simulink model "main_WU_motion"  (R2023a)
settings: Solver=VariableStepAuto  StartTime=0.0  StopTime=3.88  RelTol=1e-9  AbsTol=1e-9  EnableMultiTasking=on
values from neighbouring files (symbols this model uses):
  a_el = [r_ej,h_ej,r_ej]    [data.m]    (also in fo_python_to_matlab.m = [ax,ay,az])
  akt_GH = rand(1,13)*1    [inverse_dynamics.m]    (also in odvozeni_svaly.m = sym('akt_GH',[1 N_GH]))
  akt_ST = rand(1,13)*1    [inverse_dynamics.m]    (also in odvozeni_svaly.m = sym('akt_ST',[1 N_ST]))
  ccom = [-0.0110972, 0.00637508, 0.0541825]    [data.m]    (also in fo_python_to_matlab.m = [ccomx, ccomy, ccomz]; mm_python_to_matlab.m = [ccomx, ccomy, ccomz])
  cI = [5.75482e-05, 6.05521e-05, 1.05345e-05,-1.27405e-05, 1.65861e-05, 4.50136e-06]    [data.m]    (also in mm_python_to_matlab.m = [cixx, ciyy, cizz, cixy, ciyz, cizx])
  cont1 = [-0.083529 -0.01368 -0.098954]-scom    [data.m]    (also in fo_python_to_matlab.m = [x_cont1,y_cont1,z_cont1])
  cont2 = [-0.105456 -0.125076 -0.075251]-scom    [data.m]    (also in fo_python_to_matlab.m = [x_cont2,y_cont2,z_cont2])
  cont_params = [k_contact, eps]    [data.m]    (also in fo_python_to_matlab.m)
  Glenohumeral_F0M = str2double(table2array(GH(:,2)))'    [data.m]
  Glenohumeral_l0 = str2double(table2array(GH(:,3)))'    [data.m]
  h_ej = 0.15    [data.m]
  hcom = [0.000389382, -0.116338, -0.00231072]    [data.m]    (also in fo_python_to_matlab.m = [hcomx, hcomy, hcomz]; mm_python_to_matlab.m = [hcomx, hcomy, hcomz])
  hI = [0.00326632, 4.34807e-05, 0.00325004,-0.000136456, -1.30958e-06, -1.14964e-05]    [data.m]    (also in mm_python_to_matlab.m = [hixx, hiyy, hizz, hixy, hiyz, hizx])
  initialConditions = zeros(1,18)    [inverse_dynamics.m]
  k_contact = 0    [data.m]
  m = [0.0370005,0.12759,0.26363]    [data.m]    (also in fo_python_to_matlab.m = [c_m,s_m,h_m]; mm_python_to_matlab.m = [c_m,s_m,h_m])
  m_el = [x_ej,y_ej,z_ej]    [data.m]    (also in fo_python_to_matlab.m = [mx, my, mz])
  p = [c,k,g]    [data.m]    (also in fo_python_to_matlab.m)
  r_ej = 0.088    [data.m]
  Scapulothoracic_F0M = str2double(table2array(ST(:,2)))'    [data.m]
  Scapulothoracic_l0 = str2double(table2array(ST(:,3)))'    [data.m]
  scom = [-0.0512948, -0.0367122, -0.0430756]    [data.m]    (also in fo_python_to_matlab.m = [scomx, scomy, scomz]; mm_python_to_matlab.m = [scomx, scomy, scomz])
  sI = [0.00020065, 0.000202939, 0.000227237,-4.55661e-05, -7.53511e-05, -7.42694e-05]    [data.m]    (also in mm_python_to_matlab.m = [sixx, siyy, sizz, sixy, siyz, sizx])
  T_c = [-0.01433 0.02007 0.135535]    [data.m]    (also in fo_python_to_matlab.m = [T_cx,T_cy,T_cz]; mm_python_to_matlab.m = [T_cx,T_cy,T_cz]; odvozeni_svaly.m)
  T_d = 1e-20    [data.m]
  T_s = [-0.00955 -0.034 0.009]    [data.m]    (also in fo_python_to_matlab.m = [T_sx,T_sy,T_sz]; mm_python_to_matlab.m = [T_sx,T_sy,T_sz]; odvozeni_svaly.m)
  T_t = [0.006325 0.00693 0.025465]    [data.m]    (also in fo_python_to_matlab.m = [T_tx, T_ty, T_tz]; odvozeni_svaly.m)
  x_ej = -0.03    [data.m]
  y_ej = -0.1    [data.m]
  z_ej = 0.05    [data.m]
undefined symbols (not defined in the file or in its folder): phi_0, r_0, r_10, r_20, X, Y, Z
libraries: sm_lib x165, nesl_utility x96
(part 5 of 5)

== system main_WU_motion/scapulohumeral_rhythm/2_points_contact/ellipsoidal_joint_2 ==
  PS-Simulink Converter : nesl_utility/PS-Simulink Converter  PhysicalDomain=network_engine_domain  SubClassName=ps_output  LeftPortType=input  RightPortType=output  PseudoPeriodic=off  Frequencies=[]  VectorFormat=inherit  Unit=inherit  AffineConversion=off
  Simulink-PS Converter : nesl_utility/Simulink-PS Converter  PhysicalDomain=network_engine_domain  SubClassName=ps_input  LeftPortType=input  RightPortType=output  PseudoPeriodic=off  Frequencies=[]  NoiseDistribution=none  NoiseParameters=[]  Unit=1  AffineConversion=off  FilteringAndDerivatives=filter  SimscapeFilterOrder=2  InputFilterTimeConstant=0.001  UdotUserProvided=0
  axis : sm_lib/Joints/Revolute Joint  JointMode=Normal  SenseConstraintForce=off  SenseConstraintForceX=off  SenseConstraintForceY=off  SenseConstraintForceZ=off  SenseConstraintTorque=off  SenseConstraintTorqueX=off  SenseConstraintTorqueY=off  SenseConstraintTorqueZ=off  SenseTotalForce=off  SenseTotalForceX=off  SenseTotalForceY=off  SenseTotalForceZ=off  SenseTotalTorque=off  SenseTotalTorqueX=off  SenseTotalTorqueY=off  SenseTotalTorqueZ=off  CompositeWrenchDir=FollowerOnBase  CompositeWrenchFrame=BaseFrame  EquilibriumPosition=0  EquilibriumPositionUnits=deg  SpringStiffness=0  SpringStiffnessUnits=N*m/deg  DampingCoefficient=0  DampingCoefficientUnits=N*m/(deg/s)  TorqueActuationMode=NoTorque  MotionActuationMode=ComputedMotion  SensePosition=off  SenseVelocity=off  SenseAcceleration=off  SenseTorqueForce=off  SenseLowerLimitTorqueForce=off  SenseUpperLimitTorqueForce=off  LowerLimitSpecify=off  LowerLimitBound=-90  LowerLimitBoundUnits=deg  LowerLimitStiffness=1e4  LowerLimitStiffnessUnits=N*m/deg  LowerLimitDamping=10  LowerLimitDampingUnits=N*m/(deg/s)  LowerLimitTransitionRegionWidth=0.1  LowerLimitTransitionRegionWidthUnits=deg  UpperLimitSpecify=off  UpperLimitBound=90  UpperLimitBoundUnits=deg  UpperLimitStiffness=1e4  UpperLimitStiffnessUnits=N*m/deg  UpperLimitDamping=10  UpperLimitDampingUnits=N*m/(deg/s)  UpperLimitTransitionRegionWidth=0.1  UpperLimitTransitionRegionWidthUnits=deg  PositionTargetSpecify=on  PositionTargetPriority=High  PositionTargetValue=phi_20  PositionTargetValueUnits=rad  VelocityTargetSpecify=on  VelocityTargetPriority=High  VelocityTargetValue=0  VelocityTargetValueUnits=rad/s
  delay_r : TransportDelay  DelayTime=T_d  InitialOutput=r_20
  h : sm_lib/Joints/Prismatic Joint  JointMode=Normal  SenseConstraintForce=off  SenseConstraintForceX=off  SenseConstraintForceY=off  SenseConstraintForceZ=off  SenseConstraintTorque=off  SenseConstraintTorqueX=off  SenseConstraintTorqueY=off  SenseConstraintTorqueZ=off  SenseTotalForce=off  SenseTotalForceX=off  SenseTotalForceY=off  SenseTotalForceZ=off  SenseTotalTorque=off  SenseTotalTorqueX=off  SenseTotalTorqueY=off  SenseTotalTorqueZ=off  CompositeWrenchDir=FollowerOnBase  CompositeWrenchFrame=BaseFrame  EquilibriumPosition=0  EquilibriumPositionUnits=m  SpringStiffness=0  SpringStiffnessUnits=N/m  DampingCoefficient=0  DampingCoefficientUnits=N/(m/s)  TorqueActuationMode=NoTorque  MotionActuationMode=ComputedMotion  SensePosition=on  SenseVelocity=off  SenseAcceleration=off  SenseTorqueForce=off  SenseLowerLimitTorqueForce=off  SenseUpperLimitTorqueForce=off  LowerLimitSpecify=on  LowerLimitBound=h_min  LowerLimitBoundUnits=m  LowerLimitStiffness=1e6  LowerLimitStiffnessUnits=N/m  LowerLimitDamping=1e3  LowerLimitDampingUnits=N/(m/s)  LowerLimitTransitionRegionWidth=1e-4  LowerLimitTransitionRegionWidthUnits=m  UpperLimitSpecify=on  UpperLimitBound=h_max  UpperLimitBoundUnits=m  UpperLimitStiffness=1e6  UpperLimitStiffnessUnits=N/m  UpperLimitDamping=1e3  UpperLimitDampingUnits=N/(m/s)  UpperLimitTransitionRegionWidth=1e-4  UpperLimitTransitionRegionWidthUnits=m  PositionTargetSpecify=on  PositionTargetPriority=High  PositionTargetValue=h_20  PositionTargetValueUnits=m  VelocityTargetSpecify=on  VelocityTargetPriority=High  VelocityTargetValue=0  VelocityTargetValueUnits=m/s
  r : sm_lib/Joints/Prismatic Joint  JointMode=Normal  SenseConstraintForce=off  SenseConstraintForceX=off  SenseConstraintForceY=off  SenseConstraintForceZ=off  SenseConstraintTorque=off  SenseConstraintTorqueX=off  SenseConstraintTorqueY=off  SenseConstraintTorqueZ=off  SenseTotalForce=off  SenseTotalForceX=off  SenseTotalForceY=off  SenseTotalForceZ=off  SenseTotalTorque=off  SenseTotalTorqueX=off  SenseTotalTorqueY=off  SenseTotalTorqueZ=off  CompositeWrenchDir=FollowerOnBase  CompositeWrenchFrame=BaseFrame  EquilibriumPosition=0  EquilibriumPositionUnits=m  SpringStiffness=0  SpringStiffnessUnits=N/m  DampingCoefficient=0  DampingCoefficientUnits=N/(m/s)  TorqueActuationMode=ComputedTorque  MotionActuationMode=InputMotion  SensePosition=off  SenseVelocity=off  SenseAcceleration=off  SenseTorqueForce=off  SenseLowerLimitTorqueForce=off  SenseUpperLimitTorqueForce=off  LowerLimitSpecify=off  LowerLimitBound=-1  LowerLimitBoundUnits=m  LowerLimitStiffness=1e6  LowerLimitStiffnessUnits=N/m  LowerLimitDamping=1e3  LowerLimitDampingUnits=N/(m/s)  LowerLimitTransitionRegionWidth=1e-4  LowerLimitTransitionRegionWidthUnits=m  UpperLimitSpecify=off  UpperLimitBound=1  UpperLimitBoundUnits=m  UpperLimitStiffness=1e6  UpperLimitStiffnessUnits=N/m  UpperLimitDamping=1e3  UpperLimitDampingUnits=N/(m/s)  UpperLimitTransitionRegionWidth=1e-4  UpperLimitTransitionRegionWidthUnits=m  PositionTargetSpecify=on  PositionTargetPriority=Low  PositionTargetValue=r_20  PositionTargetValueUnits=m  VelocityTargetSpecify=on  VelocityTargetPriority=Low  VelocityTargetValue=0  VelocityTargetValueUnits=m/s
  r = fcn(h) : MATLAB Function  TreatAsAtomicUnit=on
  rot_-x_90 : sm_lib/Frames and Transforms/Rigid Transform  TranslationMethod=None  TranslationStandardOffset=0  TranslationStandardOffsetUnits=m  TranslationStandardAxis=+Z  TranslationCartesianOffset=[0 0 0]  TranslationCartesianOffsetUnits=m  TranslationROffset=0  TranslationROffsetUnits=m  TranslationZOffset=0  TranslationZOffsetUnits=m  TranslationThetaOffset=0  TranslationThetaOffsetUnits=deg  RotationMethod=StandardAxis  RotationAngleUnits=deg  RotationStandardAxis=-X  RotationAngle=90  RotationArbitraryAxis=[0 0 1]  FollAlignAxisA=+X  BaseAlignAxisA=+Y  FollAlignAxisB=+Y  BaseAlignAxisB=+Z  RotationSequenceAxes=FollowerAxes  RotationSequence=XYX  RotationSequenceAngles=[0 0 0]  RotationSequenceAnglesUnits=deg  RotationMatrix=[1 0 0; 0 1 0; 0 0 1]  Quaternion=[1 0 0 0]
  rot_-y_90 : sm_lib/Frames and Transforms/Rigid Transform  TranslationMethod=None  TranslationStandardOffset=0  TranslationStandardOffsetUnits=m  TranslationStandardAxis=+Z  TranslationCartesianOffset=[0 0 0]  TranslationCartesianOffsetUnits=m  TranslationROffset=0  TranslationROffsetUnits=m  TranslationZOffset=0  TranslationZOffsetUnits=m  TranslationThetaOffset=0  TranslationThetaOffsetUnits=deg  RotationMethod=StandardAxis  RotationAngleUnits=deg  RotationStandardAxis=-Y  RotationAngle=90  RotationArbitraryAxis=[0 0 1]  FollAlignAxisA=+X  BaseAlignAxisA=+Y  FollAlignAxisB=+Y  BaseAlignAxisB=+Z  RotationSequenceAxes=FollowerAxes  RotationSequence=XYX  RotationSequenceAngles=[0 0 0]  RotationSequenceAnglesUnits=deg  RotationMatrix=[1 0 0; 0 1 0; 0 0 1]  Quaternion=[1 0 0 0]
  scp_h : Scope
  scp_r : Scope
  B : PMIOPort  Side=Left
  F : PMIOPort  Port=2  Side=Right
  wires:
  PS-Simulink Converter/1 -> r = fcn(h)/1(h), scp_h/1
  delay_r/1 -> scp_r/1, Simulink-PS Converter/1
  r = fcn(h)/1(r) -> delay_r/1
  connections:
  rot_-x_90/LConn1 -- B/RConn1
  axis/LConn1 -- rot_-x_90/RConn1
  h/RConn2 -- PS-Simulink Converter/LConn1
  Simulink-PS Converter/RConn1 -- r/LConn2
  r/LConn1 -- rot_-y_90/RConn1
  F/RConn1 -- r/RConn1
  h/RConn1 -- rot_-y_90/LConn1
  h/LConn1 -- axis/RConn1

== system main_WU_motion/scapulohumeral_rhythm/2_points_contact/tools ==
  In1 : Inport
  cartensian_X : Subsystem

== system main_WU_motion/scapulohumeral_rhythm/Subsystem/point 1 ==
  External Force and Torque : sm_lib/Forces and Torques/External Force and Torque  ForceResolutionFrame=World  EnableForceX=on  EnableForceY=on  EnableForceZ=on  EnableForce=off  TorqueResolutionFrame=AttachedFrame  EnableTorqueX=off  EnableTorqueY=off  EnableTorqueZ=off  EnableTorque=off
  F : MATLAB Function  TreatAsAtomicUnit=on
  Mux : Mux  Inputs=3
  Mux1 : Mux  Inputs=3
  PS-Simulink Converter : nesl_utility/PS-Simulink Converter  PhysicalDomain=network_engine_domain  SubClassName=ps_output  LeftPortType=input  RightPortType=output  PseudoPeriodic=off  Frequencies=[]  VectorFormat=inherit  Unit=inherit  AffineConversion=off
  PS-Simulink Converter1 : nesl_utility/PS-Simulink Converter  PhysicalDomain=network_engine_domain  SubClassName=ps_output  LeftPortType=input  RightPortType=output  PseudoPeriodic=off  Frequencies=[]  VectorFormat=inherit  Unit=inherit  AffineConversion=off
  PS-Simulink Converter2 : nesl_utility/PS-Simulink Converter  PhysicalDomain=network_engine_domain  SubClassName=ps_output  LeftPortType=input  RightPortType=output  PseudoPeriodic=off  Frequencies=[]  VectorFormat=inherit  Unit=inherit  AffineConversion=off
  "S_1 -> S" : sm_lib/Frames and Transforms/Rigid Transform  TranslationMethod=Cartesian  TranslationStandardOffset=0  TranslationStandardOffsetUnits=m  TranslationStandardAxis=+Z  TranslationCartesianOffset=cont1  TranslationCartesianOffsetUnits=m  TranslationROffset=0  TranslationROffsetUnits=m  TranslationZOffset=0  TranslationZOffsetUnits=m  TranslationThetaOffset=0  TranslationThetaOffsetUnits=deg  RotationMethod=None  RotationAngleUnits=deg  RotationStandardAxis=+Z  RotationAngle=0.0  RotationArbitraryAxis=[0 0 1]  FollAlignAxisA=+X  BaseAlignAxisA=+Y  FollAlignAxisB=+Y  BaseAlignAxisB=+Z  RotationSequenceAxes=FollowerAxes  RotationSequence=XYX  RotationSequenceAngles=[0 0 0]  RotationSequenceAnglesUnits=deg  RotationMatrix=[1 0 0; 0 1 0; 0 0 1]  Quaternion=[1 0 0 0]
  Scope : Scope
  Simulink-PS Converter : nesl_utility/Simulink-PS Converter  PhysicalDomain=network_engine_domain  SubClassName=ps_input  LeftPortType=input  RightPortType=output  PseudoPeriodic=off  Frequencies=[]  NoiseDistribution=none  NoiseParameters=[]  Unit=1  AffineConversion=off  FilteringAndDerivatives=provide  SimscapeFilterOrder=1  InputFilterTimeConstant=0.001  UdotUserProvided=0
  Simulink-PS Converter1 : nesl_utility/Simulink-PS Converter  PhysicalDomain=network_engine_domain  SubClassName=ps_input  LeftPortType=input  RightPortType=output  PseudoPeriodic=off  Frequencies=[]  NoiseDistribution=none  NoiseParameters=[]  Unit=1  AffineConversion=off  FilteringAndDerivatives=provide  SimscapeFilterOrder=1  InputFilterTimeConstant=0.001  UdotUserProvided=0
  Simulink-PS Converter2 : nesl_utility/Simulink-PS Converter  PhysicalDomain=network_engine_domain  SubClassName=ps_input  LeftPortType=input  RightPortType=output  PseudoPeriodic=off  Frequencies=[]  NoiseDistribution=none  NoiseParameters=[]  Unit=1  AffineConversion=off  FilteringAndDerivatives=provide  SimscapeFilterOrder=1  InputFilterTimeConstant=0.001  UdotUserProvided=0
  Terminator : Terminator
  Transform Sensor : sm_lib/Frames and Transforms/Transform Sensor  MeasurementFrame=World  RotationSequence=XYX  SenseAngle=off  SenseAxis=off  SenseQ=off  SenseR=off  SenseRotationSequence=off  SenseOmegaX=off  SenseOmegaY=off  SenseOmegaZ=off  SenseQDot=off  SenseRDot=off  SenseRotationSequenceDot=off  SenseAlphaX=off  SenseAlphaY=off  SenseAlphaZ=off  SenseQDDot=off  SenseRDDot=off  SenseX=on  SenseY=on  SenseZ=on  SenseRad=off  SenseAzim=off  SenseDist=off  SenseInc=off  SenseXDot=off  SenseYDot=off  SenseZDot=off  SenseRadDot=off  SenseAzimDot=off  SenseDistDot=off  SenseIncDot=off  SenseXDDot=off  SenseYDDot=off  SenseZDDot=off  SenseRadDDot=off  SenseAzimDDot=off  SenseDistDDot=off  SenseIncDDot=off
  Frame : PMIOPort  Side=Left
  Contact point1 : PMIOPort  Port=2  Side=Right
  contact point 1 force : Outport
  wires:
  PS-Simulink Converter2/1 -> Mux1/3, F/3(z)
  F/3(Fz) -> contact point 1 force/1, Simulink-PS Converter2/1, Mux/3  "z"
  PS-Simulink Converter1/1 -> Mux1/2, F/2(y)
  F/1(Fx) -> Simulink-PS Converter/1, Mux/1  "x"
  F/2(Fy) -> Simulink-PS Converter1/1, Mux/2  "y"
  PS-Simulink Converter/1 -> Mux1/1, F/1(x)
  Mux1/1 -> Scope/1
  Mux/1 -> Terminator/1
  connections:
  External Force and Torque/LConn2 -- Simulink-PS Converter1/RConn1
  Transform Sensor/RConn4 -- PS-Simulink Converter2/LConn1
  Transform Sensor/RConn2 -- PS-Simulink Converter/LConn1
  Transform Sensor/LConn1 -- Frame/RConn1
  Simulink-PS Converter/RConn1 -- External Force and Torque/LConn1
  Transform Sensor/RConn3 -- PS-Simulink Converter1/LConn1
  Simulink-PS Converter2/RConn1 -- External Force and Torque/LConn3
  External Force and Torque/RConn1 -- "S_1 -> S"/RConn1 -- Transform Sensor/RConn1
  "S_1 -> S"/LConn1 -- Contact point1/RConn1

== system main_WU_motion/scapulohumeral_rhythm/Subsystem/point 2 ==
  External Force and Torque : sm_lib/Forces and Torques/External Force and Torque  ForceResolutionFrame=World  EnableForceX=on  EnableForceY=on  EnableForceZ=on  EnableForce=off  TorqueResolutionFrame=AttachedFrame  EnableTorqueX=off  EnableTorqueY=off  EnableTorqueZ=off  EnableTorque=off
  F : MATLAB Function  TreatAsAtomicUnit=on
  Mux : Mux  Inputs=3
  Mux1 : Mux  Inputs=3
  PS-Simulink Converter : nesl_utility/PS-Simulink Converter  PhysicalDomain=network_engine_domain  SubClassName=ps_output  LeftPortType=input  RightPortType=output  PseudoPeriodic=off  Frequencies=[]  VectorFormat=inherit  Unit=inherit  AffineConversion=off
  PS-Simulink Converter1 : nesl_utility/PS-Simulink Converter  PhysicalDomain=network_engine_domain  SubClassName=ps_output  LeftPortType=input  RightPortType=output  PseudoPeriodic=off  Frequencies=[]  VectorFormat=inherit  Unit=inherit  AffineConversion=off
  PS-Simulink Converter2 : nesl_utility/PS-Simulink Converter  PhysicalDomain=network_engine_domain  SubClassName=ps_output  LeftPortType=input  RightPortType=output  PseudoPeriodic=off  Frequencies=[]  VectorFormat=inherit  Unit=inherit  AffineConversion=off
  "S_2 -> S" : sm_lib/Frames and Transforms/Rigid Transform  TranslationMethod=Cartesian  TranslationStandardOffset=0  TranslationStandardOffsetUnits=m  TranslationStandardAxis=+Z  TranslationCartesianOffset=cont2  TranslationCartesianOffsetUnits=m  TranslationROffset=0  TranslationROffsetUnits=m  TranslationZOffset=0  TranslationZOffsetUnits=m  TranslationThetaOffset=0  TranslationThetaOffsetUnits=deg  RotationMethod=None  RotationAngleUnits=deg  RotationStandardAxis=+Z  RotationAngle=0.0  RotationArbitraryAxis=[0 0 1]  FollAlignAxisA=+X  BaseAlignAxisA=+Y  FollAlignAxisB=+Y  BaseAlignAxisB=+Z  RotationSequenceAxes=FollowerAxes  RotationSequence=XYX  RotationSequenceAngles=[0 0 0]  RotationSequenceAnglesUnits=deg  RotationMatrix=[1 0 0; 0 1 0; 0 0 1]  Quaternion=[1 0 0 0]
  Scope : Scope
  Simulink-PS Converter : nesl_utility/Simulink-PS Converter  PhysicalDomain=network_engine_domain  SubClassName=ps_input  LeftPortType=input  RightPortType=output  PseudoPeriodic=off  Frequencies=[]  NoiseDistribution=none  NoiseParameters=[]  Unit=1  AffineConversion=off  FilteringAndDerivatives=provide  SimscapeFilterOrder=1  InputFilterTimeConstant=0.001  UdotUserProvided=0
  Simulink-PS Converter1 : nesl_utility/Simulink-PS Converter  PhysicalDomain=network_engine_domain  SubClassName=ps_input  LeftPortType=input  RightPortType=output  PseudoPeriodic=off  Frequencies=[]  NoiseDistribution=none  NoiseParameters=[]  Unit=1  AffineConversion=off  FilteringAndDerivatives=provide  SimscapeFilterOrder=1  InputFilterTimeConstant=0.001  UdotUserProvided=0
  Simulink-PS Converter2 : nesl_utility/Simulink-PS Converter  PhysicalDomain=network_engine_domain  SubClassName=ps_input  LeftPortType=input  RightPortType=output  PseudoPeriodic=off  Frequencies=[]  NoiseDistribution=none  NoiseParameters=[]  Unit=1  AffineConversion=off  FilteringAndDerivatives=provide  SimscapeFilterOrder=1  InputFilterTimeConstant=0.001  UdotUserProvided=0
  Transform Sensor : sm_lib/Frames and Transforms/Transform Sensor  MeasurementFrame=World  RotationSequence=XYX  SenseAngle=off  SenseAxis=off  SenseQ=off  SenseR=off  SenseRotationSequence=off  SenseOmegaX=off  SenseOmegaY=off  SenseOmegaZ=off  SenseQDot=off  SenseRDot=off  SenseRotationSequenceDot=off  SenseAlphaX=off  SenseAlphaY=off  SenseAlphaZ=off  SenseQDDot=off  SenseRDDot=off  SenseX=on  SenseY=on  SenseZ=on  SenseRad=off  SenseAzim=off  SenseDist=off  SenseInc=off  SenseXDot=off  SenseYDot=off  SenseZDot=off  SenseRadDot=off  SenseAzimDot=off  SenseDistDot=off  SenseIncDot=off  SenseXDDot=off  SenseYDDot=off  SenseZDDot=off  SenseRadDDot=off  SenseAzimDDot=off  SenseDistDDot=off  SenseIncDDot=off
  Frame : PMIOPort  Side=Left
  Contact point : PMIOPort  Port=2  Side=Right
  contact point 2 force : Outport
  wires:
  PS-Simulink Converter/1 -> F/1(x), Mux1/1
  F/2(Fy) -> Mux/2, Simulink-PS Converter1/1  "y"
  F/1(Fx) -> Mux/1, Simulink-PS Converter/1  "x"
  PS-Simulink Converter1/1 -> F/2(y), Mux1/2
  Mux/1 -> contact point 2 force/1
  F/3(Fz) -> Mux/3, Simulink-PS Converter2/1  "z"
  PS-Simulink Converter2/1 -> F/3(z), Mux1/3
  Mux1/1 -> Scope/1
  connections:
  Transform Sensor/RConn1 -- "S_2 -> S"/RConn1 -- External Force and Torque/RConn1
  Simulink-PS Converter2/RConn1 -- External Force and Torque/LConn3
  Transform Sensor/RConn3 -- PS-Simulink Converter1/LConn1
  Simulink-PS Converter/RConn1 -- External Force and Torque/LConn1
  Transform Sensor/LConn1 -- Frame/RConn1
  Transform Sensor/RConn2 -- PS-Simulink Converter/LConn1
  Transform Sensor/RConn4 -- PS-Simulink Converter2/LConn1
  External Force and Torque/LConn2 -- Simulink-PS Converter1/RConn1
  "S_2 -> S"/LConn1 -- Contact point/RConn1

== system main_WU_motion/scapulohumeral_rhythm/2_points_contact/tools/cartensian_X ==
  Mux : Mux  Inputs=3
  PS-Simulink Converter : nesl_utility/PS-Simulink Converter  PhysicalDomain=network_engine_domain  SubClassName=ps_output  LeftPortType=input  RightPortType=output  PseudoPeriodic=off  Frequencies=[]  VectorFormat=inherit  Unit=inherit  AffineConversion=off
  PS-Simulink Converter1 : nesl_utility/PS-Simulink Converter  PhysicalDomain=network_engine_domain  SubClassName=ps_output  LeftPortType=input  RightPortType=output  PseudoPeriodic=off  Frequencies=[]  VectorFormat=inherit  Unit=inherit  AffineConversion=off
  PS-Simulink Converter2 : nesl_utility/PS-Simulink Converter  PhysicalDomain=network_engine_domain  SubClassName=ps_output  LeftPortType=input  RightPortType=output  PseudoPeriodic=off  Frequencies=[]  VectorFormat=inherit  Unit=inherit  AffineConversion=off
  To Workspace : ToWorkspace  VariableName=X  SampleTime=-1
  Transform Sensor : sm_lib/Frames and Transforms/Transform Sensor  MeasurementFrame=World  RotationSequence=XYX  SenseAngle=off  SenseAxis=off  SenseQ=off  SenseR=off  SenseRotationSequence=off  SenseOmegaX=off  SenseOmegaY=off  SenseOmegaZ=off  SenseQDot=off  SenseRDot=off  SenseRotationSequenceDot=off  SenseAlphaX=off  SenseAlphaY=off  SenseAlphaZ=off  SenseQDDot=off  SenseRDDot=off  SenseX=on  SenseY=on  SenseZ=on  SenseRad=off  SenseAzim=off  SenseDist=off  SenseInc=off  SenseXDot=off  SenseYDot=off  SenseZDot=off  SenseRadDot=off  SenseAzimDot=off  SenseDistDot=off  SenseIncDot=off  SenseXDDot=off  SenseYDDot=off  SenseZDDot=off  SenseRadDDot=off  SenseAzimDDot=off  SenseDistDDot=off  SenseIncDDot=off
  World Frame : sm_lib/Frames and Transforms/World Frame
  X : PMIOPort  Side=Left
  wires:
  PS-Simulink Converter/1 -> Mux/1
  Mux/1 -> To Workspace/1
  PS-Simulink Converter1/1 -> Mux/2
  PS-Simulink Converter2/1 -> Mux/3
  connections:
  Transform Sensor/RConn4 -- PS-Simulink Converter2/LConn1
  Transform Sensor/RConn2 -- PS-Simulink Converter/LConn1
  PS-Simulink Converter1/LConn1 -- Transform Sensor/RConn3
  Transform Sensor/RConn1 -- X/RConn1
  World Frame/RConn1 -- Transform Sensor/LConn1

== matlab function main_WU_motion/MATLAB Function ==
  data: t input; q input; dq input; ddq input; m parameter; y output; cI parameter; sI parameter; hI parameter; ccom parameter; scom parameter; hcom parameter; T_c parameter; T_s parameter; p parameter; T_t parameter; m_el parameter; a_el parameter; cont1 parameter; cont2 parameter; cont_params parameter; akt_GH parameter; Glenohumeral_F0M parameter; Glenohumeral_l0 parameter; akt_ST parameter; Scapulothoracic_F0M parameter; Scapulothoracic_l0 parameter
function y = fcn(t,q,dq,ddq,m,cI,sI,hI,ccom,scom,hcom,T_c,T_s,p,T_t, m_el, a_el, cont1, cont2, cont_params,akt_GH, Glenohumeral_F0M, Glenohumeral_l0,akt_ST, Scapulothoracic_F0M, Scapulothoracic_l0)
y = zeros(18,1);
y = fcn_ID(t,q,dq,ddq,m,cI,sI,hI,ccom,scom,hcom,T_t,T_c,T_s,p,m_el,a_el,cont1,cont2,cont_params,akt_GH,-Glenohumeral_F0M, Glenohumeral_l0,akt_ST,-Scapulothoracic_F0M,Scapulothoracic_l0);

== matlab function main_WU_motion/MATLAB Function1 ==
  data: u input; y output; p_coords parameter
function y = fcn(u,p_coords)
y = zeros(9,1);
% for i=1:9
%     y(i) = polyval(p_coords(i,:),u);
%     % y(i) = 45*cos(u)-45;
% end

== matlab function main_WU_motion/scapulohumeral_rhythm/1_point_contact/r = fcn(h) ==
  data: h input; r output; h_ej parameter; r_ej parameter
function r = fcn(h,h_ej,r_ej)

r = sqrt((r_ej^2)*(1-h^2/h_ej^2));

== matlab function main_WU_motion/scapulohumeral_rhythm/2_points_contact/ellipsoidal_joint_1/r = fcn(h) ==
  data: h input; r output; h_ej parameter; r_ej parameter
function r = fcn(h,h_ej,r_ej)

r = sqrt((r_ej^2)*(1-h^2/h_ej^2));

== matlab function main_WU_motion/scapulohumeral_rhythm/2_points_contact/ellipsoidal_joint_2/r = fcn(h) ==
  data: h input; r output; h_ej parameter; r_ej parameter
function r = fcn(h,h_ej,r_ej)

r = sqrt((r_ej^2)*(1-h^2/h_ej^2));

== matlab function main_WU_motion/glenohumeral_muscles/INFRSP/Active_factor_norm ==
  data: Fa_norm output; lm input; l0 input; a input
function Fa_norm = fcn(lm,l0,a)
f_gauss = 0.25;
Fa_norm = (exp(-(lm/l0-1)^2/f_gauss))*a;

== matlab function main_WU_motion/glenohumeral_muscles/INFRSP/Passive_force_norm ==
  data: lm input; Fp_norm output; l0 input
function Fp_norm = fcn(lm,l0)
Fp_norm = ((lm/l0)^3)*exp(8*lm/l0-12.9);

== matlab function main_WU_motion/glenohumeral_muscles/LAT/Active_factor_norm ==
  data: Fa_norm output; lm input; l0 input; a input
function Fa_norm = fcn(lm,l0,a)
f_gauss = 0.25;
Fa_norm = (exp(-(lm/l0-1)^2/f_gauss))*a;

== matlab function main_WU_motion/glenohumeral_muscles/LAT/Passive_force_norm ==
  data: lm input; Fp_norm output; l0 input
function Fp_norm = fcn(lm,l0)
Fp_norm = ((lm/l0)^3)*exp(8*lm/l0-12.9);

== matlab function main_WU_motion/glenohumeral_muscles/PECM1/Active_factor_norm ==
  data: Fa_norm output; lm input; l0 input; a input
function Fa_norm = fcn(lm,l0,a)
f_gauss = 0.25;
Fa_norm = (exp(-(lm/l0-1)^2/f_gauss))*a;

== matlab function main_WU_motion/glenohumeral_muscles/PECM1/Passive_force_norm ==
  data: lm input; Fp_norm output; l0 input
function Fp_norm = fcn(lm,l0)
Fp_norm = ((lm/l0)^3)*exp(8*lm/l0-12.9);

== matlab function main_WU_motion/glenohumeral_muscles/PECM2/Active_factor_norm ==
  data: Fa_norm output; lm input; l0 input; a input
function Fa_norm = fcn(lm,l0,a)
f_gauss = 0.25;
Fa_norm = (exp(-(lm/l0-1)^2/f_gauss))*a;

== matlab function main_WU_motion/glenohumeral_muscles/PECM2/Passive_force_norm ==
  data: lm input; Fp_norm output; l0 input
function Fp_norm = fcn(lm,l0)
Fp_norm = ((lm/l0)^3)*exp(8*lm/l0-12.9);

== matlab function main_WU_motion/glenohumeral_muscles/PECM3/Active_factor_norm ==
  data: Fa_norm output; lm input; l0 input; a input
function Fa_norm = fcn(lm,l0,a)
f_gauss = 0.25;
Fa_norm = (exp(-(lm/l0-1)^2/f_gauss))*a;

== matlab function main_WU_motion/glenohumeral_muscles/PECM3/Passive_force_norm ==
  data: lm input; Fp_norm output; l0 input
function Fp_norm = fcn(lm,l0)
Fp_norm = ((lm/l0)^3)*exp(8*lm/l0-12.9);

== matlab function main_WU_motion/glenohumeral_muscles/SUBSC/Active_factor_norm ==
  data: Fa_norm output; lm input; l0 input; a input
function Fa_norm = fcn(lm,l0,a)
f_gauss = 0.25;
Fa_norm = (exp(-(lm/l0-1)^2/f_gauss))*a;

== matlab function main_WU_motion/glenohumeral_muscles/SUBSC/Passive_force_norm ==
  data: lm input; Fp_norm output; l0 input
function Fp_norm = fcn(lm,l0)
Fp_norm = ((lm/l0)^3)*exp(8*lm/l0-12.9);

== matlab function main_WU_motion/glenohumeral_muscles/SUPSP/Active_factor_norm ==
  data: Fa_norm output; lm input; l0 input; a input
function Fa_norm = fcn(lm,l0,a)
f_gauss = 0.25;
Fa_norm = (exp(-(lm/l0-1)^2/f_gauss))*a;

== matlab function main_WU_motion/glenohumeral_muscles/CORB/Active_factor_norm ==
  data: Fa_norm output; lm input; l0 input; a input
function Fa_norm = fcn(lm,l0,a)
f_gauss = 0.25;
Fa_norm = (exp(-(lm/l0-1)^2/f_gauss))*a;

== matlab function main_WU_motion/glenohumeral_muscles/CORB/Passive_force_norm ==
  data: lm input; Fp_norm output; l0 input
function Fp_norm = fcn(lm,l0)
Fp_norm = ((lm/l0)^3)*exp(8*lm/l0-12.9);

== matlab function main_WU_motion/glenohumeral_muscles/SUPSP/Passive_force_norm ==
  data: lm input; Fp_norm output; l0 input
function Fp_norm = fcn(lm,l0)
Fp_norm = ((lm/l0)^3)*exp(8*lm/l0-12.9);

== matlab function main_WU_motion/glenohumeral_muscles/TMAJ/Active_factor_norm ==
  data: Fa_norm output; lm input; l0 input; a input
function Fa_norm = fcn(lm,l0,a)
f_gauss = 0.25;
Fa_norm = (exp(-(lm/l0-1)^2/f_gauss))*a;

== matlab function main_WU_motion/glenohumeral_muscles/TMAJ/Passive_force_norm ==
  data: lm input; Fp_norm output; l0 input
function Fp_norm = fcn(lm,l0)
Fp_norm = ((lm/l0)^3)*exp(8*lm/l0-12.9);

== matlab function main_WU_motion/glenohumeral_muscles/TMIN/Active_factor_norm ==
  data: Fa_norm output; lm input; l0 input; a input
function Fa_norm = fcn(lm,l0,a)
f_gauss = 0.25;
Fa_norm = (exp(-(lm/l0-1)^2/f_gauss))*a;

== matlab function main_WU_motion/glenohumeral_muscles/TMIN/Passive_force_norm ==
  data: lm input; Fp_norm output; l0 input
function Fp_norm = fcn(lm,l0)
Fp_norm = ((lm/l0)^3)*exp(8*lm/l0-12.9);

== matlab function main_WU_motion/scapulothoracic_muscles/SBCL/Active_factor_norm ==
  data: Fa_norm output; lm input; l0 input; a input
function Fa_norm = fcn(lm,l0,a)
f_gauss = 0.25;
Fa_norm = (exp(-(lm/l0-1)^2/f_gauss))*a;

== matlab function main_WU_motion/scapulothoracic_muscles/SBCL/Passive_force_norm ==
  data: lm input; Fp_norm output; l0 input
function Fp_norm = fcn(lm,l0)
Fp_norm = ((lm/l0)^3)*exp(8*lm/l0-12.9);

== matlab function main_WU_motion/scapulothoracic_muscles/SRA1/Active_factor_norm ==
  data: Fa_norm output; lm input; l0 input; a input
function Fa_norm = fcn(lm,l0,a)
f_gauss = 0.25;
Fa_norm = (exp(-(lm/l0-1)^2/f_gauss))*a;

== matlab function main_WU_motion/scapulothoracic_muscles/SRA1/Passive_force_norm ==
  data: lm input; Fp_norm output; l0 input
function Fp_norm = fcn(lm,l0)
Fp_norm = ((lm/l0)^3)*exp(8*lm/l0-12.9);

== matlab function main_WU_motion/scapulothoracic_muscles/SRA2/Active_factor_norm ==
  data: Fa_norm output; lm input; l0 input; a input
function Fa_norm = fcn(lm,l0,a)
f_gauss = 0.25;
Fa_norm = (exp(-(lm/l0-1)^2/f_gauss))*a;

== matlab function main_WU_motion/scapulothoracic_muscles/SRA2/Passive_force_norm ==
  data: lm input; Fp_norm output; l0 input
function Fp_norm = fcn(lm,l0)
Fp_norm = ((lm/l0)^3)*exp(8*lm/l0-12.9);

== matlab function main_WU_motion/scapulothoracic_muscles/SRA3/Active_factor_norm ==
  data: Fa_norm output; lm input; l0 input; a input
function Fa_norm = fcn(lm,l0,a)
f_gauss = 0.25;
Fa_norm = (exp(-(lm/l0-1)^2/f_gauss))*a;

== matlab function main_WU_motion/scapulothoracic_muscles/SRA3/Passive_force_norm ==
  data: lm input; Fp_norm output; l0 input
function Fp_norm = fcn(lm,l0)
Fp_norm = ((lm/l0)^3)*exp(8*lm/l0-12.9);

== matlab function main_WU_motion/scapulothoracic_muscles/TRP1/Active_factor_norm ==
  data: Fa_norm output; lm input; l0 input; a input
function Fa_norm = fcn(lm,l0,a)
f_gauss = 0.25;
Fa_norm = (exp(-(lm/l0-1)^2/f_gauss))*a;

== matlab function main_WU_motion/scapulothoracic_muscles/TRP1/Passive_force_norm ==
  data: lm input; Fp_norm output; l0 input
function Fp_norm = fcn(lm,l0)
Fp_norm = ((lm/l0)^3)*exp(8*lm/l0-12.9);

== matlab function main_WU_motion/scapulothoracic_muscles/TRP2/Active_factor_norm ==
  data: Fa_norm output; lm input; l0 input; a input
function Fa_norm = fcn(lm,l0,a)
f_gauss = 0.25;
Fa_norm = (exp(-(lm/l0-1)^2/f_gauss))*a;

== matlab function main_WU_motion/scapulothoracic_muscles/LVS/Active_factor_norm ==
  data: Fa_norm output; lm input; l0 input; a input
function Fa_norm = fcn(lm,l0,a)
f_gauss = 0.25;
Fa_norm = (exp(-(lm/l0-1)^2/f_gauss))*a;

== matlab function main_WU_motion/glenohumeral_muscles/DELT1/Active_factor_norm ==
  data: Fa_norm output; lm input; l0 input; a input
function Fa_norm = fcn(lm,l0,a)
f_gauss = 0.25;
Fa_norm = (exp(-(lm/l0-1)^2/f_gauss))*a;

== matlab function main_WU_motion/scapulothoracic_muscles/LVS/Passive_force_norm ==
  data: lm input; Fp_norm output; l0 input
function Fp_norm = fcn(lm,l0)
Fp_norm = ((lm/l0)^3)*exp(8*lm/l0-12.9);

== matlab function main_WU_motion/scapulothoracic_muscles/RMN/Active_factor_norm ==
  data: Fa_norm output; lm input; l0 input; a input
function Fa_norm = fcn(lm,l0,a)
f_gauss = 0.25;
Fa_norm = (exp(-(lm/l0-1)^2/f_gauss))*a;

== matlab function main_WU_motion/scapulothoracic_muscles/RMN/Passive_force_norm ==
  data: lm input; Fp_norm output; l0 input
function Fp_norm = fcn(lm,l0)
Fp_norm = ((lm/l0)^3)*exp(8*lm/l0-12.9);

== matlab function main_WU_motion/scapulothoracic_muscles/RMNJ1/Active_factor_norm ==
  data: Fa_norm output; lm input; l0 input; a input
function Fa_norm = fcn(lm,l0,a)
f_gauss = 0.25;
Fa_norm = (exp(-(lm/l0-1)^2/f_gauss))*a;

== matlab function main_WU_motion/scapulothoracic_muscles/RMNJ1/Passive_force_norm ==
  data: lm input; Fp_norm output; l0 input
function Fp_norm = fcn(lm,l0)
Fp_norm = ((lm/l0)^3)*exp(8*lm/l0-12.9);

== matlab function main_WU_motion/scapulothoracic_muscles/RMNJ2/Active_factor_norm ==
  data: Fa_norm output; lm input; l0 input; a input
function Fa_norm = fcn(lm,l0,a)
f_gauss = 0.25;
Fa_norm = (exp(-(lm/l0-1)^2/f_gauss))*a;

== matlab function main_WU_motion/scapulothoracic_muscles/RMNJ2/Passive_force_norm ==
  data: lm input; Fp_norm output; l0 input
function Fp_norm = fcn(lm,l0)
Fp_norm = ((lm/l0)^3)*exp(8*lm/l0-12.9);

== matlab function main_WU_motion/scapulothoracic_muscles/PMN/Active_factor_norm ==
  data: Fa_norm output; lm input; l0 input; a input
function Fa_norm = fcn(lm,l0,a)
f_gauss = 0.25;
Fa_norm = (exp(-(lm/l0-1)^2/f_gauss))*a;

== matlab function main_WU_motion/scapulothoracic_muscles/PMN/Passive_force_norm ==
  data: lm input; Fp_norm output; l0 input
function Fp_norm = fcn(lm,l0)
Fp_norm = ((lm/l0)^3)*exp(8*lm/l0-12.9);

== matlab function main_WU_motion/scapulothoracic_muscles/TRP2/Passive_force_norm ==
  data: lm input; Fp_norm output; l0 input
function Fp_norm = fcn(lm,l0)
Fp_norm = ((lm/l0)^3)*exp(8*lm/l0-12.9);

== matlab function main_WU_motion/scapulothoracic_muscles/TRP3/Active_factor_norm ==
  data: Fa_norm output; lm input; l0 input; a input
function Fa_norm = fcn(lm,l0,a)
f_gauss = 0.25;
Fa_norm = (exp(-(lm/l0-1)^2/f_gauss))*a;

== matlab function main_WU_motion/scapulohumeral_rhythm/1_point_contact/phi = fcn(h) ==
  data: h input; phi output; h_ej parameter; r_ej parameter
function phi = fcn(h,h_ej,r_ej)

phi = atan(-(r_ej*h)/(h_ej^2*sqrt(1-h^2/h_ej^2)));

== matlab function main_WU_motion/scapulohumeral_rhythm/Subsystem/point 1/F ==
  data: x input; Fx output; y input; z input; Fy output; Fz output; x_ej parameter; y_ej parameter; z_ej parameter; r_ej parameter; h_ej parameter; eps parameter; k_contact parameter
function [Fx,Fy,Fz]= fcn(x,y,z,x_ej, y_ej, z_ej, r_ej, h_ej, eps, k_contact)

f = ((x-x_ej)/r_ej)^2+((y-y_ej)/h_ej)^2+((z-z_ej)/r_ej)^2-1;
F = 1/2*(f-sqrt(f^2+eps^2));

Fx = -k_contact*(x-x_ej)*(r_ej^2+h_ej^2+r_ej^2)/(r_ej^2)*F;
Fy = -k_contact*(y-y_ej)*(r_ej^2+h_ej^2+r_ej^2)/(h_ej^2)*F;
Fz = -k_contact*(z-z_ej)*(r_ej^2+h_ej^2+r_ej^2)/(r_ej^2)*F;

%% 2D
% 
% f = ((x-mx)/ax)^2+((z-mz)/az)^2-1;
% F = 1/2*(f-sqrt(f^2+eps^2));
% 
% Fx = -k*(x-mx)*(ax^2+ay^2)/(ax^2)*F;
% Fy = -k*(y-my)*(ax^2+ay^2)/(ay^2)*F;
% Fz = -k*(z-mz)*(ax^2+ay^2)/(az^2)*F;

== matlab function main_WU_motion/scapulohumeral_rhythm/Subsystem/point 2/F ==
  data: x input; Fx output; y input; z input; Fy output; Fz output; x_ej parameter; y_ej parameter; z_ej parameter; r_ej parameter; h_ej parameter; eps parameter; k_contact parameter
function [Fx,Fy,Fz]= fcn(x,y,z,x_ej, y_ej, z_ej, r_ej, h_ej, eps, k_contact)

f = ((x-x_ej)/r_ej)^2+((y-y_ej)/h_ej)^2+((z-z_ej)/r_ej)^2-1;
F = 1/2*(f-sqrt(f^2+eps^2));

Fx = -k_contact*(x-x_ej)*(r_ej^2+h_ej^2+r_ej^2)/(r_ej^2)*F;
Fy = -k_contact*(y-y_ej)*(r_ej^2+h_ej^2+r_ej^2)/(h_ej^2)*F;
Fz = -k_contact*(z-z_ej)*(r_ej^2+h_ej^2+r_ej^2)/(r_ej^2)*F;

%% 2D
% 
% f = ((x-mx)/ax)^2+((z-mz)/az)^2-1;
% F = 1/2*(f-sqrt(f^2+eps^2));
% 
% Fx = -k*(x-mx)*(ax^2+ay^2)/(ax^2)*F;
% Fy = -k*(y-my)*(ax^2+ay^2)/(ay^2)*F;
% Fz = -k*(z-mz)*(ax^2+ay^2)/(az^2)*F;

== matlab function main_WU_motion/scapulothoracic_muscles/TRP3/Passive_force_norm ==
  data: lm input; Fp_norm output; l0 input
function Fp_norm = fcn(lm,l0)
Fp_norm = ((lm/l0)^3)*exp(8*lm/l0-12.9);

== matlab function main_WU_motion/scapulothoracic_muscles/TRP4/Active_factor_norm ==
  data: Fa_norm output; lm input; l0 input; a input
function Fa_norm = fcn(lm,l0,a)
f_gauss = 0.25;
Fa_norm = (exp(-(lm/l0-1)^2/f_gauss))*a;

== matlab function main_WU_motion/scapulothoracic_muscles/TRP4/Passive_force_norm ==
  data: lm input; Fp_norm output; l0 input
function Fp_norm = fcn(lm,l0)
Fp_norm = ((lm/l0)^3)*exp(8*lm/l0-12.9);

== matlab function main_WU_motion/glenohumeral_muscles/DELT1/Passive_force_norm ==
  data: lm input; Fp_norm output; l0 input
function Fp_norm = fcn(lm,l0)
Fp_norm = ((lm/l0)^3)*exp(8*lm/l0-12.9);

== matlab function main_WU_motion/glenohumeral_muscles/DELT2/Passive_force_norm ==
  data: lm input; Fp_norm output; l0 input
function Fp_norm = fcn(lm,l0)
Fp_norm = ((lm/l0)^3)*exp(8*lm/l0-12.9);

== matlab function main_WU_motion/glenohumeral_muscles/DELT3/Active_factor_norm ==
  data: Fa_norm output; lm input; l0 input; a input
function Fa_norm = fcn(lm,l0,a)
f_gauss = 0.25;
Fa_norm = (exp(-(lm/l0-1)^2/f_gauss))*a;

== matlab function main_WU_motion/glenohumeral_muscles/DELT3/Passive_force_norm ==
  data: lm input; Fp_norm output; l0 input
function Fp_norm = fcn(lm,l0)
Fp_norm = ((lm/l0)^3)*exp(8*lm/l0-12.9);

== matlab function main_WU_motion/glenohumeral_muscles/DELT2/Active_factor_norm ==
  data: Fa_norm output; lm input; l0 input; a input
function Fa_norm = fcn(lm,l0,a)
f_gauss = 0.25;
Fa_norm = (exp(-(lm/l0-1)^2/f_gauss))*a;
